simulink model "driving_dynamics_model"  (R2018b)
settings: Solver=VariableStepAuto  StartTime=0.0  StopTime=10.0  RelTol=1e-3
PreLoadFcn:
  | AtSourceModelPreLoad(bdroot);
PostLoadFcn:
  | AtSourceModelPostLoad(bdroot);
InitFcn:
  | AtSourceModelInit(bdroot,0);
values from neighbouring files (symbols this model uses):
  a = 1.8    [formulacar_params.mat]    (also in longitudinal_coefficients.m; roadcar_params.mat = 1.1)
  A = 1.25    [formulacar_params.mat]    (also in longitudinal_coefficients.m; roadcar_params.mat = 1.8)
  a1 = -1e-5    (= -1e-05)    [longitudinal_coefficients.m]
  a2 = 1.25    [longitudinal_coefficients.m]
  B = 4.1576    [longitudinal_coefficients.m]
  C = 1.7180    (= 1.718)    [longitudinal_coefficients.m]
  cd = 0.4    [longitudinal_coefficients.m]
  cz = 1    [formulacar_params.mat]    (also in longitudinal_coefficients.m; roadcar_params.mat = 0)
  g = 9.81    [formulacar_params.mat]    (also in longitudinal_coefficients.m; quarter_car_model_parameters.m; roadcar_params.mat)
  h = 0.2    [longitudinal_coefficients.m]
  Iwheel = 0.9    [longitudinal_coefficients.m]
  L = 3.5    [formulacar_params.mat]    (also in longitudinal_coefficients.m; roadcar_params.mat = 2.8)
  m = 850    [formulacar_params.mat]    (also in longitudinal_coefficients.m; roadcar_params.mat = 1650)
  r = 0.375    [longitudinal_coefficients.m]
  rho = 1.225    [formulacar_params.mat]    (also in longitudinal_coefficients.m; roadcar_params.mat)
undefined symbols (not defined in the file or in its folder): enginemap, enginerpm, rpm_idling, rpm_limit, rpm_shift, rpm_up, Tengmax, throttlepos
settings Model: Creator=Cassio.Freitas  LastModifiedBy=Cassio.Freitas

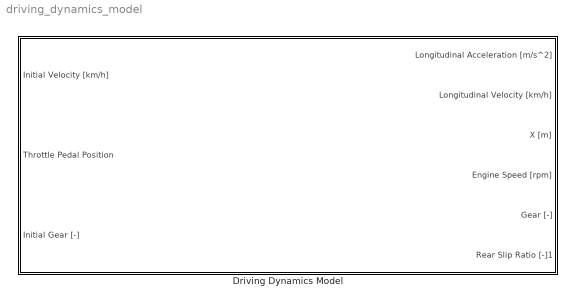
== system driving_dynamics_model ==
  "Driving Dynamics Model " : Subsystem

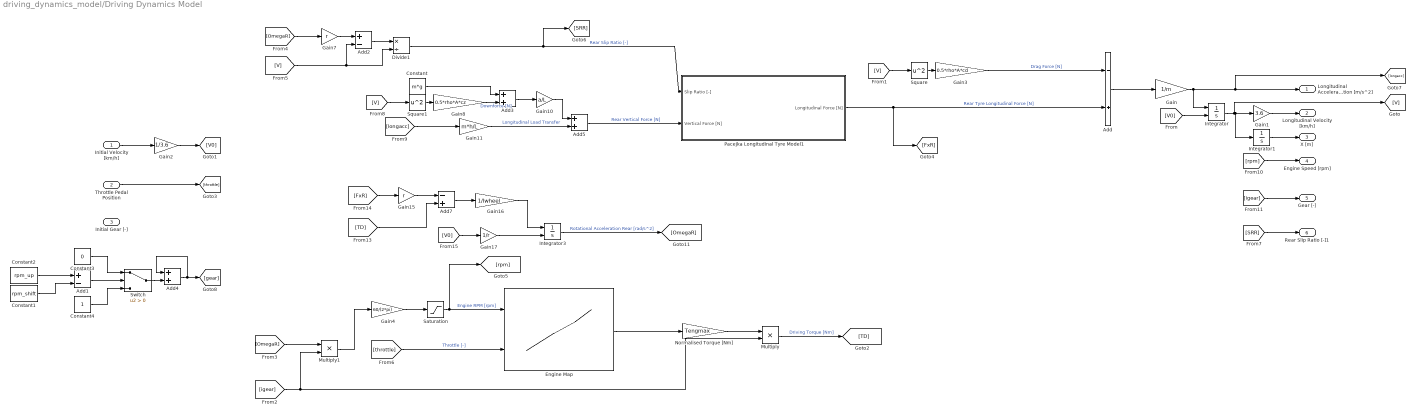
== system driving_dynamics_model/Driving Dynamics Model  ==
  Initial Velocity [km/h] : Inport
  Throttle Pedal Position : Inport  Port=2
  Initial Gear [-] : Inport  Port=3
  Add : Sum  Inputs=-+
  Add1 : Sum  Inputs=+-
  Add2 : Sum  Inputs=+-
  Add3 : Sum
  Add4 : Sum
  Add5 : Sum
  Add7 : Sum  Inputs=-+
  Constant : Constant  Value=m*g
  Constant1 : Constant  Value=rpm_shift
  Constant2 : Constant  Value=rpm_up
  Constant3 : Constant  Value=0
  Constant4 : Constant
  Divide1 : Product  Inputs=*/
  Engine Map : Lookup_n-D  BreakpointsForDimension1=enginerpm  BreakpointsForDimension2=throttlepos  Table=enginemap  InternalRulePriority=Speed  RndMeth=Simplest  InputSameDT=on
  Gain : Gain  Gain=1/m
  Gain1 : Gain  Gain=3.6
  Gain10 : Gain  Gain=a/L
  Gain11 : Gain  Gain=m*h/L
  Gain15 : Gain  Gain=r
  Gain16 : Gain  Gain=1/Iwheel
  Gain17 : Gain  Gain=1/r
  Gain2 : Gain  Gain=1/3.6
  Gain3 : Gain  Gain=0.5*rho*A*cd
  Gain4 : Gain  Gain=60/(2*pi)
  Gain7 : Gain  Gain=r
  Gain8 : Gain  Gain=0.5*rho*A*cz
  Integrator : Integrator  InitialConditionSource=external
  Integrator1 : Integrator
  Integrator3 : Integrator  InitialConditionSource=external
  Multiply : Product
  Multiply1 : Product
  "Normalised Torque [Nm] " : Gain  Gain=Tengmax
  Pacejka Longitudinal Tyre Model1 : Subsystem
  Saturation : Saturate  UpperLimit=rpm_limit  LowerLimit=rpm_idling
  Square : Math  Operator=square  SaturateOnIntegerOverflow=on
  Square1 : Math  Operator=square  SaturateOnIntegerOverflow=on
  Switch : Switch  Criteria=u2 > Threshold
  Longitudinal Acceleration [m/s^2] : Outport
  Longitudinal Velocity [km/h] : Outport  Port=2
  X [m] : Outport  Port=3
  Engine Speed [rpm] : Outport  Port=4
  Gear [-] : Outport  Port=5
  Rear Slip Ratio [-]1 : Outport  Port=6
  wires:
  Gain3/1 -> Add/1  "Drag Force [N]"
  [longacc] -> Gain11/1
  Gain17/1 -> Integrator3/2
  Gain8/1 -> Add3/2  "Downforce [N]"
  Gain2/1 -> [V0]
  Throttle Pedal Position/1 -> [throttle]
  [V] -> Square/1
  Gain15/1 -> Add7/1
  Square/1 -> Gain3/1
  [V] -> Square1/1
  [FxR] -> Gain15/1
  Add7/1 -> Gain16/1
  Add5/1 -> Pacejka Longitudinal Tyre Model1/2(Vertical Force [N])  "Rear Vertical Force [N]"
  Integrator3/1 -> [OmegaR]  "Rotational Acceleration Rear [rad/s^2]"
  [V0] -> Gain17/1
  Add/1 -> Gain/1
  Initial Velocity [km/h]/1 -> Gain2/1
  [OmegaR] -> Gain7/1
  Divide1/1 -> [SRR], Pacejka Longitudinal Tyre Model1/1(Slip Ratio [-])  "Rear Slip Ratio [-]"
  Constant/1 -> Add3/1
  Gain11/1 -> Add5/2  "Longitudinal Load Transfer"
  Integrator1/1 -> X [m]/1
  Pacejka Longitudinal Tyre Model1/1(Longitudinal Force [N]) -> Add/2, [FxR]  "Rear Tyre Longitudinal Force [N]"
  Add3/1 -> Gain10/1
  Integrator/1 -> [V], Integrator1/1, Gain1/1
  Gain7/1 -> Add2/1
  Add2/1 -> Divide1/1
  Square1/1 -> Gain8/1
  [V] -> Add2/2, Divide1/2
  Gain16/1 -> Integrator3/1
  Gain1/1 -> Longitudinal Velocity [km/h]/1
  [TD] -> Add7/2
  [V0] -> Integrator/2
  Gain/1 -> Integrator/1, [longacc], Longitudinal Acceleration [m/s^2]/1
  [SRR] -> Rear Slip Ratio [-]1/1
  Gain10/1 -> Add5/1
  "Normalised Torque [Nm] "/1 -> Multiply/1
  [igear] -> Multiply1/2, Multiply/2
  Multiply/1 -> [TD]  "Driving Torque [Nm]"
  Engine Map/1 -> "Normalised Torque [Nm] "/1
  [throttle] -> Engine Map/2  "Throttle [-]"
  [OmegaR] -> Multiply1/1
  Gain4/1 -> Saturation/1
  Multiply1/1 -> Gain4/1
  [rpm] -> Engine Speed [rpm]/1
  [igear] -> Gear [-]/1
  Saturation/1 -> [rpm], Engine Map/1  "Engine RPM [rpm]"
  Constant2/1 -> Add1/1
  Constant1/1 -> Add1/2
  Add1/1 -> Switch/2
  Constant3/1 -> Switch/1
  Constant4/1 -> Switch/3
  Switch/1 -> Add4/2
  Add4/1 -> [gear], Add4/1

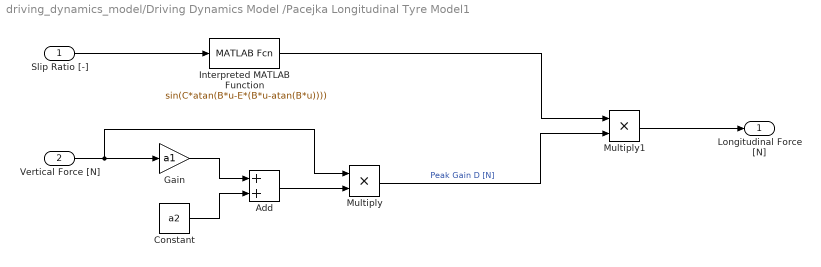
== system driving_dynamics_model/Driving Dynamics Model /Pacejka Longitudinal Tyre Model1 ==
  Slip Ratio [-] : Inport
  Vertical Force [N] : Inport  Port=2
  Add : Sum
  Constant : Constant  Value=a2
  Gain : Gain  Gain=a1
  Interpreted MATLAB Function : MATLABFcn  MATLABFcn=sin(C*atan(B*u-E*(B*u-atan(B*u))))
  Multiply : Product
  Multiply1 : Product
  Longitudinal Force [N] : Outport
  wires:
  Vertical Force [N]/1 -> Multiply/1, Gain/1
  Constant/1 -> Add/2
  Gain/1 -> Add/1
  Add/1 -> Multiply/2
  Multiply/1 -> Multiply1/2  "Peak Gain D [N]"
  Slip Ratio [-]/1 -> Interpreted MATLAB Function/1
  Interpreted MATLAB Function/1 -> Multiply1/1
  Multiply1/1 -> Longitudinal Force [N]/1
